simulink model "Robot_1"  (R2023b)
settings: Solver=VariableStepAuto  StartTime=0.0  StopTime=10.0  RelTol=1e-3
settings Model: DataDictionary=Robot_1DD.sldd  Creator=maxju  LastModifiedBy=maxju

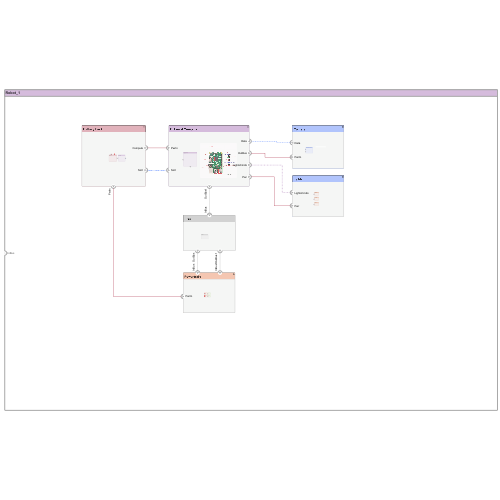
[thumbnail: Simulink's stored preview of the top-level diagram]
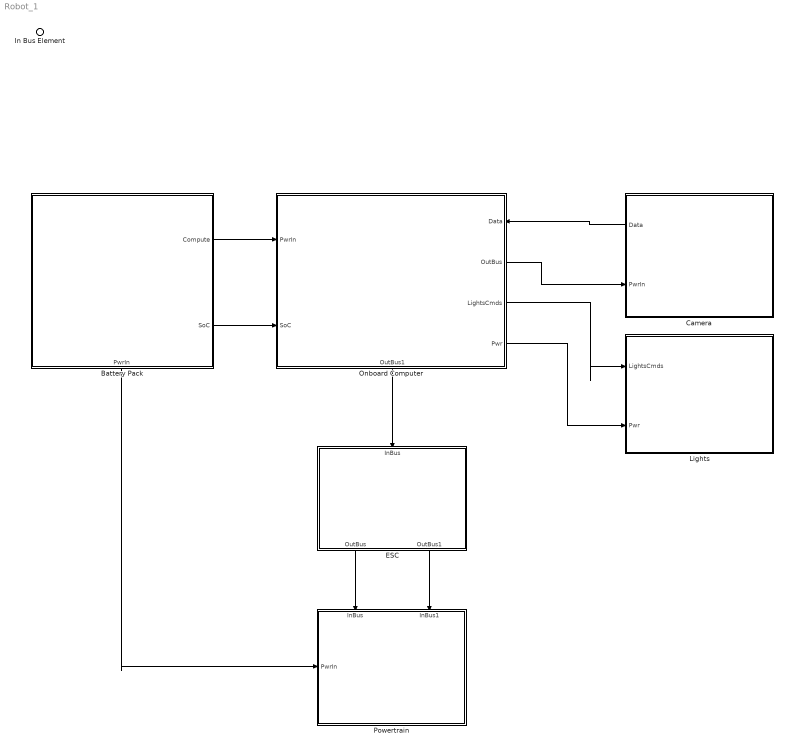
== system Robot_1 ==
  In Bus Element : Inport  PortName=InBus
  Battery Pack : Subsystem
      settings: PortSchema="{\"entries\":[{\"content\":{\"headerSize\":26,\"margin\":15,\"minimumSpacing\":25,\"sides\":[{\"content\":{},\"type\":\"ConnectorPlacement.EquallySpacedRectSide\",\"uuid\":\"346f2912-6369-49a7-a9f0-29be96ed2aab\"},{\"content\":{\"connectorIds\":[\"Out1\",\"Out2\"],\"side\":\"RIGHT\"},\"type\":\"ConnectorPlacement.EquallySpacedRectSide\",\"uuid\":\"c8393630-96ba-47a0-be32-8aed75641cc7\"},{\"content\":{\"side\":\"TOP\"},\"type\":\"ConnectorPlacement.EquallySpacedRectSide\",\"uuid\":\"3ed129fe-5e63-4396-9170-1d52c5d32d40\"},{\"content\":{\"connectorIds\":[\"Out3\"],\"side\":\"BOTTOM\"},\"type\":\"ConnectorPlacement.EquallySpacedRectSide\",\"uuid\":\"1c04906c-6323-40fc-a7b2-3d731de826fc\"}]},\"type\":\"ConnectorPlacement.EquallySpacedConnector\",\"uuid\":\"219e7a86-40fe-4101-a52d-fba84ff528a7\"}],\"packageUris\":[\"http://schema.mathworks.com/mf0/Connector/R2020b\"],\"version\":\"1.0\"}"
  Camera : Subsystem
      settings: PortSchema="{\"entries\":[{\"content\":{\"headerSize\":26,\"margin\":15,\"minimumSpacing\":25,\"sides\":[{\"content\":{\"connectorIds\":[\"Out1\",\"In1\"]},\"type\":\"ConnectorPlacement.EquallySpacedRectSide\",\"uuid\":\"0e3134fb-fb1a-4646-97ad-e2d6271ac93c\"},{\"content\":{\"side\":\"RIGHT\"},\"type\":\"ConnectorPlacement.EquallySpacedRectSide\",\"uuid\":\"f6782e40-1403-4bf9-a42f-252b6616eef0\"},{\"content\":{\"side\":\"TOP\"},\"type\":\"ConnectorPlacement.EquallySpacedRectSide\",\"uuid\":\"161a9c94-3c0d-4f4d-984f-997aeb99b9b4\"}]},\"type\":\"ConnectorPlacement.EquallySpacedConnector\",\"uuid\":\"22acbad8-3a60-4658-bd61-aa1d6af050b7\"}],\"packageUris\":[\"http://schema.mathworks.com/mf0/Connector/R2020b\"],\"version\":\"1.0\"}"
  ESC : Subsystem
      settings: PortSchema="{\"entries\":[{\"content\":{\"headerSize\":26,\"margin\":15,\"minimumSpacing\":25,\"sides\":[{\"content\":{},\"type\":\"ConnectorPlacement.EquallySpacedRectSide\",\"uuid\":\"1141339f-839f-42a9-af72-07ea182886c4\"},{\"content\":{\"side\":\"RIGHT\"},\"type\":\"ConnectorPlacement.EquallySpacedRectSide\",\"uuid\":\"dbe82220-b0cd-4347-8409-f18d181432e5\"},{\"content\":{\"connectorIds\":[\"In1\"],\"side\":\"TOP\"},\"type\":\"ConnectorPlacement.EquallySpacedRectSide\",\"uuid\":\"b87040ad-d69b-40eb-96a3-a12b59f8261a\"},{\"content\":{\"connectorIds\":[\"Out1\",\"Out2\"],\"side\":\"BOTTOM\"},\"type\":\"ConnectorPlacement.EquallySpacedRectSide\",\"uuid\":\"a37703f8-e732-485f-af8e-5cc2f63c328a\"}]},\"type\":\"ConnectorPlacement.EquallySpacedConnector\",\"uuid\":\"cd1bc216-bb56-48d6-9fa3-a849dd38b660\"}],\"packageUris\":[\"http://schema.mathworks.com/mf0/Connector/R2020b\"],\"version\":\"1.0\"}"
  Lights : Subsystem
      settings: PortSchema="{\"entries\":[{\"content\":{\"headerSize\":26,\"margin\":15,\"minimumSpacing\":25,\"sides\":[{\"content\":{\"connectorIds\":[\"In1\",\"In2\"]},\"type\":\"ConnectorPlacement.EquallySpacedRectSide\",\"uuid\":\"346f2912-6369-49a7-a9f0-29be96ed2aab\"},{\"content\":{\"side\":\"RIGHT\"},\"type\":\"ConnectorPlacement.EquallySpacedRectSide\",\"uuid\":\"c8393630-96ba-47a0-be32-8aed75641cc7\"},{\"content\":{\"side\":\"TOP\"},\"type\":\"ConnectorPlacement.EquallySpacedRectSide\",\"uuid\":\"3ed129fe-5e63-4396-9170-1d52c5d32d40\"}]},\"type\":\"ConnectorPlacement.EquallySpacedConnector\",\"uuid\":\"219e7a86-40fe-4101-a52d-fba84ff528a7\"}],\"packageUris\":[\"http://schema.mathworks.com/mf0/Connector/R2020b\"],\"version\":\"1.0\"}"
  Onboard Computer : Subsystem
      settings: PortSchema="{\"entries\":[{\"content\":{\"headerSize\":26,\"margin\":15,\"minimumSpacing\":25,\"sides\":[{\"content\":{\"connectorIds\":[\"In3\",\"In2\"]},\"type\":\"ConnectorPlacement.EquallySpacedRectSide\",\"uuid\":\"346f2912-6369-49a7-a9f0-29be96ed2aab\"},{\"content\":{\"connectorIds\":[\"In1\",\"Out2\",\"Out3\",\"Out4\"],\"side\":\"RIGHT\"},\"type\":\"ConnectorPlacement.EquallySpacedRectSide\",\"uuid\":\"c8393630-96ba-47a0-be32-8aed75641cc7\"},{\"content\":{\"side\":\"TOP\"},\"type\":\"ConnectorPlacement.EquallySpacedRectSide\",\"uuid\":\"3ed129fe-5e63-4396-9170-1d52c5d32d40\"},{\"content\":{\"connectorIds\":[\"Out1\"],\"side\":\"BOTTOM\"},\"type\":\"ConnectorPlacement.EquallySpacedRectSide\",\"uuid\":\"e427383b-7eca-4773-95c8-b4eaaf910589\"}]},\"type\":\"ConnectorPlacement.EquallySpacedConnector\",\"uuid\":\"219e7a86-40fe-4101-a52d-fba84ff528a7\"}],\"packageUris\":[\"http://schema.mathworks.com/mf0/Connector/R2020b\"],\"version\":\"1.0\"}"
  Powertrain : Subsystem
      settings: PortSchema="{\"entries\":[{\"content\":{\"headerSize\":26,\"margin\":15,\"minimumSpacing\":25,\"sides\":[{\"content\":{\"connectorIds\":[\"In3\"]},\"type\":\"ConnectorPlacement.EquallySpacedRectSide\",\"uuid\":\"0e3134fb-fb1a-4646-97ad-e2d6271ac93c\"},{\"content\":{\"side\":\"RIGHT\"},\"type\":\"ConnectorPlacement.EquallySpacedRectSide\",\"uuid\":\"f6782e40-1403-4bf9-a42f-252b6616eef0\"},{\"content\":{\"connectorIds\":[\"In1\",\"In2\"],\"side\":\"TOP\"},\"type\":\"ConnectorPlacement.EquallySpacedRectSide\",\"uuid\":\"161a9c94-3c0d-4f4d-984f-997aeb99b9b4\"},{\"content\":{\"side\":\"BOTTOM\"},\"type\":\"ConnectorPlacement.EquallySpacedRectSide\",\"uuid\":\"0cc85a08-61c2-4dc1-a2c9-a661b3276f19\"}]},\"type\":\"ConnectorPlacement.EquallySpacedConnector\",\"uuid\":\"22acbad8-3a60-4658-bd61-aa1d6af050b7\"}],\"packageUris\":[\"http://schema.mathworks.com/mf0/Connector/R2020b\"],\"version\":\"1.0\"}"
  wires:
  Onboard Computer/1(OutBus1) -> ESC/1(InBus)
  Onboard Computer/3(LightsCmds) -> Lights/1(LightsCmds)
  Onboard Computer/4(Pwr) -> Lights/2(Pwr)
  Onboard Computer/2(OutBus) -> Camera/1(PwrIn)
  Battery Pack/3(PwrIn) -> Powertrain/3(PwrIn)
  Camera/1(Data) -> Onboard Computer/1(Data)
  Battery Pack/1(Compute) -> Onboard Computer/3(PwrIn)
  Battery Pack/2(SoC) -> Onboard Computer/2(SoC)
  ESC/1(OutBus) -> Powertrain/1(InBus)
  ESC/2(OutBus1) -> Powertrain/2(InBus1)

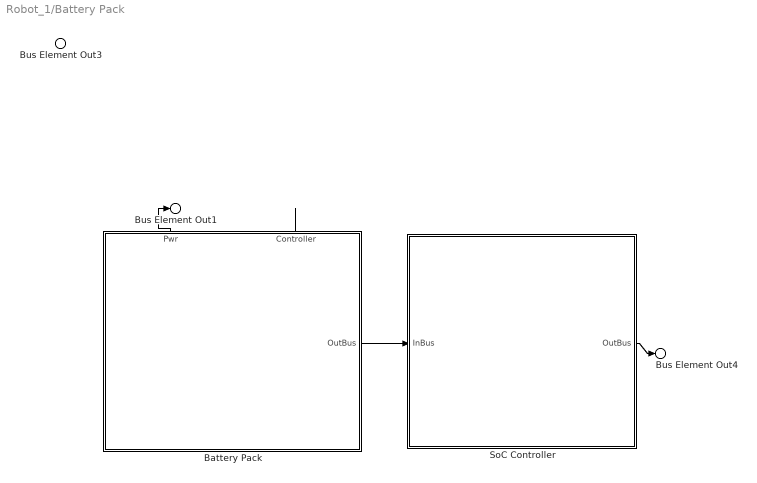
== system Robot_1/Battery Pack ==
  Battery Pack : Subsystem
      settings: PortSchema="{\"entries\":[{\"content\":{\"headerSize\":26,\"margin\":15,\"minimumSpacing\":25,\"sides\":[{\"content\":{},\"type\":\"ConnectorPlacement.EquallySpacedRectSide\",\"uuid\":\"346f2912-6369-49a7-a9f0-29be96ed2aab\"},{\"content\":{\"connectorIds\":[\"Out3\"],\"side\":\"RIGHT\"},\"type\":\"ConnectorPlacement.EquallySpacedRectSide\",\"uuid\":\"c8393630-96ba-47a0-be32-8aed75641cc7\"},{\"content\":{\"connectorIds\":[\"Out1\",\"Out2\"],\"side\":\"TOP\"},\"type\":\"ConnectorPlacement.EquallySpacedRectSide\",\"uuid\":\"3ed129fe-5e63-4396-9170-1d52c5d32d40\"},{\"content\":{\"side\":\"BOTTOM\"},\"type\":\"ConnectorPlacement.EquallySpacedRectSide\",\"uuid\":\"2c97d9a6-c0a8-4633-a49e-90eaf43f5ab4\"}]},\"type\":\"ConnectorPlacement.EquallySpacedConnector\",\"uuid\":\"219e7a86-40fe-4101-a52d-fba84ff528a7\"}],\"packageUris\":[\"http://schema.mathworks.com/mf0/Connector/R2020b\"],\"version\":\"1.0\"}"
  SoC Controller : Subsystem
      settings: PortSchema="{\"entries\":[{\"content\":{\"headerSize\":26,\"margin\":15,\"minimumSpacing\":25,\"sides\":[{\"content\":{\"connectorIds\":[\"In1\"]},\"type\":\"ConnectorPlacement.EquallySpacedRectSide\",\"uuid\":\"cf2231e3-4af8-4ed0-b91c-09d727a3483e\"},{\"content\":{\"connectorIds\":[\"Out1\"],\"side\":\"RIGHT\"},\"type\":\"ConnectorPlacement.EquallySpacedRectSide\",\"uuid\":\"4a4a1d2b-b1e3-400a-adf5-58c88c5da874\"},{\"content\":{\"side\":\"TOP\"},\"type\":\"ConnectorPlacement.EquallySpacedRectSide\",\"uuid\":\"6ce22e2e-ca4b-49c4-85bb-19d8dcc1c047\"}]},\"type\":\"ConnectorPlacement.EquallySpacedConnector\",\"uuid\":\"a895a3e5-be82-4b5e-962f-7a3c361a4de2\"}],\"packageUris\":[\"http://schema.mathworks.com/mf0/Connector/R2020b\"],\"version\":\"1.0\"}"
  Bus Element Out1 : Outport  PortName=Compute  Element=Pwr12V
  Bus Element Out4 : Outport  Port=2  PortName=SoC
  Bus Element Out3 : Outport  Port=3  PortName=PwrIn
  wires:
  Battery Pack/3(OutBus) -> SoC Controller/1(InBus)
  SoC Controller/1(OutBus) -> Bus Element Out4/1
  Battery Pack/1(Pwr) -> Bus Element Out1/1
  Battery Pack/2(Controller) -> ?

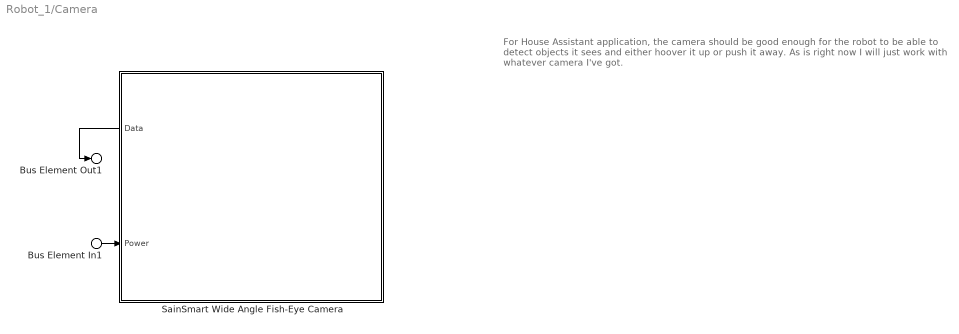
== system Robot_1/Camera ==
  note: For House Assistant application, the camera should be good enough for the robot to be able to detect objects it sees and either hoover it up or push it away.
      | As is right now I will just work with whatever camera I've got.
  Bus Element In1 : Inport  PortName=PwrIn  Element=Pwr6V
  SainSmart Wide Angle Fish-Eye Camera : Subsystem
      settings: PortSchema="{\"entries\":[{\"content\":{\"headerSize\":26,\"margin\":15,\"minimumSpacing\":25,\"sides\":[{\"content\":{\"connectorIds\":[\"Out1\",\"In1\"]},\"type\":\"ConnectorPlacement.EquallySpacedRectSide\",\"uuid\":\"0e3134fb-fb1a-4646-97ad-e2d6271ac93c\"},{\"content\":{\"side\":\"RIGHT\"},\"type\":\"ConnectorPlacement.EquallySpacedRectSide\",\"uuid\":\"f6782e40-1403-4bf9-a42f-252b6616eef0\"},{\"content\":{\"side\":\"TOP\"},\"type\":\"ConnectorPlacement.EquallySpacedRectSide\",\"uuid\":\"161a9c94-3c0d-4f4d-984f-997aeb99b9b4\"}]},\"type\":\"ConnectorPlacement.EquallySpacedConnector\",\"uuid\":\"22acbad8-3a60-4658-bd61-aa1d6af050b7\"}],\"packageUris\":[\"http://schema.mathworks.com/mf0/Connector/R2020b\"],\"version\":\"1.0\"}"
  Bus Element Out1 : Outport  PortName=Data
  wires:
  Bus Element In1/1 -> SainSmart Wide Angle Fish-Eye Camera/1(Power)
  SainSmart Wide Angle Fish-Eye Camera/1(Data) -> Bus Element Out1/1

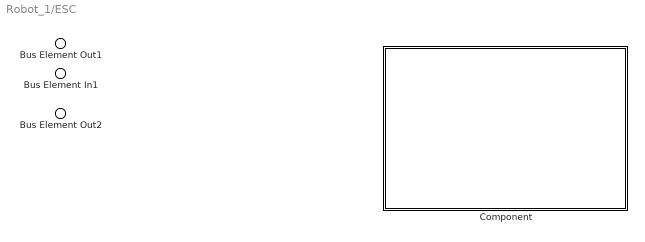
== system Robot_1/ESC ==
  Bus Element In1 : Inport  PortName=InBus
  Component : Subsystem
      settings: PortSchema="{\"entries\":[{\"content\":{\"headerSize\":26,\"margin\":15,\"minimumSpacing\":25,\"sides\":[{\"content\":{},\"type\":\"ConnectorPlacement.EquallySpacedRectSide\",\"uuid\":\"7bd470fa-bce1-4c44-a3a7-0ed7fedee971\"},{\"content\":{\"side\":\"RIGHT\"},\"type\":\"ConnectorPlacement.EquallySpacedRectSide\",\"uuid\":\"b20f4573-2099-47e2-9b7d-c115428c8e1f\"},{\"content\":{\"side\":\"TOP\"},\"type\":\"ConnectorPlacement.EquallySpacedRectSide\",\"uuid\":\"6fe36d19-1289-4062-bd44-05b1c708d213\"}]},\"type\":\"ConnectorPlacement.EquallySpacedConnector\",\"uuid\":\"3a440cc7-8cbc-4545-9d2b-44ca326050ac\"}],\"packageUris\":[\"http://schema.mathworks.com/mf0/Connector/R2020b\"],\"version\":\"1.0\"}"
  Bus Element Out1 : Outport  PortName=OutBus
  Bus Element Out2 : Outport  Port=2  PortName=OutBus1

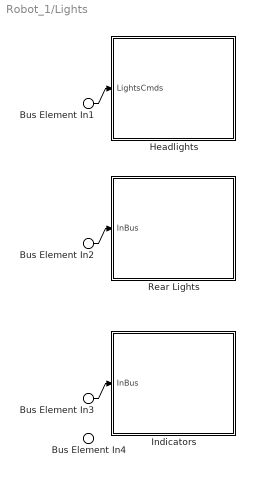
== system Robot_1/Lights ==
  Bus Element In1 : Inport  PortName=LightsCmds  Element=HeadlightsCmds
  Bus Element In2 : Inport  PortName=LightsCmds  Element=RearLightsCmds
  Bus Element In3 : Inport  PortName=LightsCmds  Element=IndicatorsCmds
  Bus Element In4 : Inport  Port=2  PortName=Pwr
  Headlights : Subsystem
      settings: PortSchema="{\"entries\":[{\"content\":{\"headerSize\":26,\"margin\":15,\"minimumSpacing\":25,\"sides\":[{\"content\":{\"connectorIds\":[\"In1\"]},\"type\":\"ConnectorPlacement.EquallySpacedRectSide\",\"uuid\":\"346f2912-6369-49a7-a9f0-29be96ed2aab\"},{\"content\":{\"side\":\"RIGHT\"},\"type\":\"ConnectorPlacement.EquallySpacedRectSide\",\"uuid\":\"c8393630-96ba-47a0-be32-8aed75641cc7\"},{\"content\":{\"side\":\"TOP\"},\"type\":\"ConnectorPlacement.EquallySpacedRectSide\",\"uuid\":\"3ed129fe-5e63-4396-9170-1d52c5d32d40\"}]},\"type\":\"ConnectorPlacement.EquallySpacedConnector\",\"uuid\":\"219e7a86-40fe-4101-a52d-fba84ff528a7\"}],\"packageUris\":[\"http://schema.mathworks.com/mf0/Connector/R2020b\"],\"version\":\"1.0\"}"
  Indicators : Subsystem
      settings: PortSchema="{\"entries\":[{\"content\":{\"headerSize\":26,\"margin\":15,\"minimumSpacing\":25,\"sides\":[{\"content\":{\"connectorIds\":[\"In1\"]},\"type\":\"ConnectorPlacement.EquallySpacedRectSide\",\"uuid\":\"346f2912-6369-49a7-a9f0-29be96ed2aab\"},{\"content\":{\"side\":\"RIGHT\"},\"type\":\"ConnectorPlacement.EquallySpacedRectSide\",\"uuid\":\"c8393630-96ba-47a0-be32-8aed75641cc7\"},{\"content\":{\"side\":\"TOP\"},\"type\":\"ConnectorPlacement.EquallySpacedRectSide\",\"uuid\":\"3ed129fe-5e63-4396-9170-1d52c5d32d40\"}]},\"type\":\"ConnectorPlacement.EquallySpacedConnector\",\"uuid\":\"219e7a86-40fe-4101-a52d-fba84ff528a7\"}],\"packageUris\":[\"http://schema.mathworks.com/mf0/Connector/R2020b\"],\"version\":\"1.0\"}"
  Rear Lights : Subsystem
      settings: PortSchema="{\"entries\":[{\"content\":{\"headerSize\":26,\"margin\":15,\"minimumSpacing\":25,\"sides\":[{\"content\":{\"connectorIds\":[\"In1\"]},\"type\":\"ConnectorPlacement.EquallySpacedRectSide\",\"uuid\":\"346f2912-6369-49a7-a9f0-29be96ed2aab\"},{\"content\":{\"side\":\"RIGHT\"},\"type\":\"ConnectorPlacement.EquallySpacedRectSide\",\"uuid\":\"c8393630-96ba-47a0-be32-8aed75641cc7\"},{\"content\":{\"side\":\"TOP\"},\"type\":\"ConnectorPlacement.EquallySpacedRectSide\",\"uuid\":\"3ed129fe-5e63-4396-9170-1d52c5d32d40\"}]},\"type\":\"ConnectorPlacement.EquallySpacedConnector\",\"uuid\":\"219e7a86-40fe-4101-a52d-fba84ff528a7\"}],\"packageUris\":[\"http://schema.mathworks.com/mf0/Connector/R2020b\"],\"version\":\"1.0\"}"
  wires:
  Bus Element In1/1 -> Headlights/1(LightsCmds)
  Bus Element In2/1 -> Rear Lights/1(InBus)
  Bus Element In3/1 -> Indicators/1(InBus)

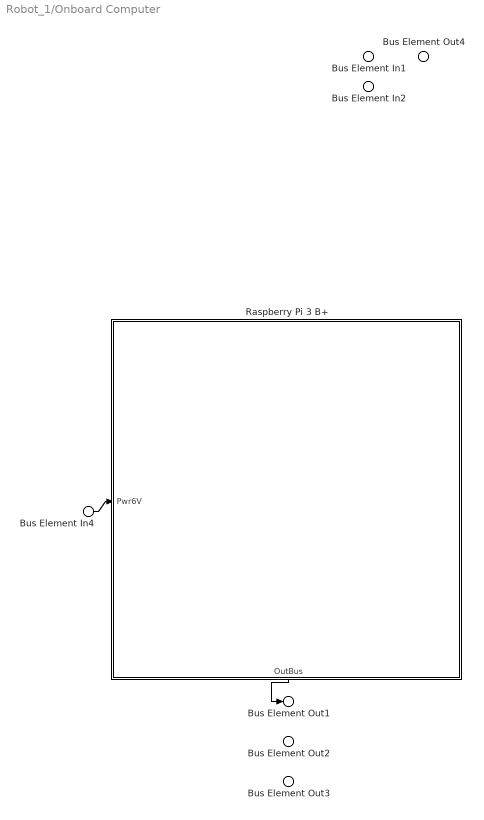
== system Robot_1/Onboard Computer ==
  Bus Element In1 : Inport  PortName=Data
  Bus Element In2 : Inport  Port=2  PortName=SoC
  Bus Element In4 : Inport  Port=3  PortName=PwrIn  Element=Pwr12V
  Raspberry Pi 3 B+ : Stateflow chart  TreatAsAtomicUnit=on
      settings: PortSchema="{\"entries\":[{\"content\":{\"headerSize\":26,\"margin\":15,\"minimumSpacing\":25,\"sides\":[{\"content\":{\"connectorIds\":[\"In1\"]},\"type\":\"ConnectorPlacement.EquallySpacedRectSide\",\"uuid\":\"0e3134fb-fb1a-4646-97ad-e2d6271ac93c\"},{\"content\":{\"side\":\"RIGHT\"},\"type\":\"ConnectorPlacement.EquallySpacedRectSide\",\"uuid\":\"f6782e40-1403-4bf9-a42f-252b6616eef0\"},{\"content\":{\"side\":\"TOP\"},\"type\":\"ConnectorPlacement.EquallySpacedRectSide\",\"uuid\":\"161a9c94-3c0d-4f4d-984f-997aeb99b9b4\"},{\"content\":{\"connectorIds\":[\"Out1\"],\"side\":\"BOTTOM\"},\"type\":\"ConnectorPlacement.EquallySpacedRectSide\",\"uuid\":\"bf1e25a0-eb6f-4642-8c09-fa933b1d8126\"}]},\"type\":\"ConnectorPlacement.EquallySpacedConnector\",\"uuid\":\"22acbad8-3a60-4658-bd61-aa1d6af050b7\"}],\"packageUris\":[\"http://schema.mathworks.com/mf0/Connector/R2020b\"],\"version\":\"1.0\"}"
  Bus Element Out4 : Outport  PortName=OutBus1
  Bus Element Out1 : Outport  Port=2  PortName=OutBus  Element=Pwr6V
  Bus Element Out2 : Outport  Port=3  PortName=LightsCmds
  Bus Element Out3 : Outport  Port=4  PortName=Pwr
  wires:
  Bus Element In4/1 -> Raspberry Pi 3 B+/1(Pwr6V)
  Raspberry Pi 3 B+/1(OutBus) -> Bus Element Out1/1

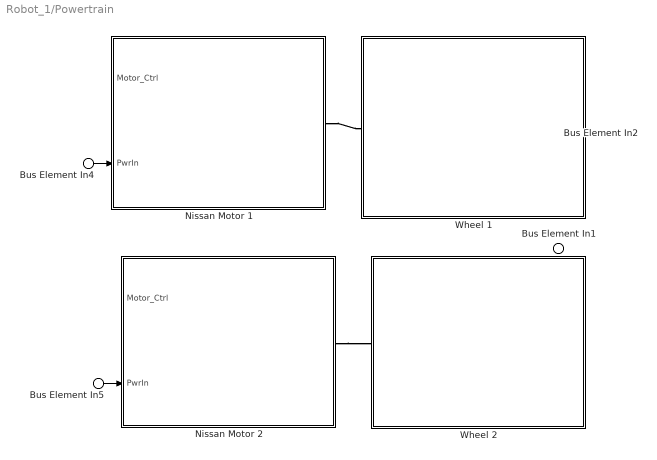
== system Robot_1/Powertrain ==
  Bus Element In1 : Inport  PortName=InBus
  Bus Element In2 : Inport  Port=2  PortName=InBus1
  Bus Element In4 : Inport  Port=3  PortName=PwrIn
  Bus Element In5 : Inport  Port=3  PortName=PwrIn
  Nissan Motor 1 : Subsystem
      settings: PortSchema="{\"entries\":[{\"content\":{\"headerSize\":26,\"margin\":15,\"minimumSpacing\":25,\"sides\":[{\"content\":{\"connectorIds\":[\"In1\",\"In2\"]},\"type\":\"ConnectorPlacement.EquallySpacedRectSide\",\"uuid\":\"346f2912-6369-49a7-a9f0-29be96ed2aab\"},{\"content\":{\"connectorIds\":[\"RConn1\"],\"side\":\"RIGHT\"},\"type\":\"ConnectorPlacement.EquallySpacedRectSide\",\"uuid\":\"c8393630-96ba-47a0-be32-8aed75641cc7\"},{\"content\":{\"side\":\"TOP\"},\"type\":\"ConnectorPlacement.EquallySpacedRectSide\",\"uuid\":\"3ed129fe-5e63-4396-9170-1d52c5d32d40\"}]},\"type\":\"ConnectorPlacement.EquallySpacedConnector\",\"uuid\":\"219e7a86-40fe-4101-a52d-fba84ff528a7\"}],\"packageUris\":[\"http://schema.mathworks.com/mf0/Connector/R2020b\"],\"version\":\"1.0\"}"
  Nissan Motor 2 : Subsystem
      settings: PortSchema="{\"entries\":[{\"content\":{\"headerSize\":26,\"margin\":15,\"minimumSpacing\":25,\"sides\":[{\"content\":{\"connectorIds\":[\"In1\",\"In2\"]},\"type\":\"ConnectorPlacement.EquallySpacedRectSide\",\"uuid\":\"346f2912-6369-49a7-a9f0-29be96ed2aab\"},{\"content\":{\"connectorIds\":[\"RConn1\"],\"side\":\"RIGHT\"},\"type\":\"ConnectorPlacement.EquallySpacedRectSide\",\"uuid\":\"c8393630-96ba-47a0-be32-8aed75641cc7\"},{\"content\":{\"side\":\"TOP\"},\"type\":\"ConnectorPlacement.EquallySpacedRectSide\",\"uuid\":\"3ed129fe-5e63-4396-9170-1d52c5d32d40\"}]},\"type\":\"ConnectorPlacement.EquallySpacedConnector\",\"uuid\":\"219e7a86-40fe-4101-a52d-fba84ff528a7\"}],\"packageUris\":[\"http://schema.mathworks.com/mf0/Connector/R2020b\"],\"version\":\"1.0\"}"
  Wheel 1 : Subsystem
      settings: PortSchema="{\"entries\":[{\"content\":{\"headerSize\":26,\"margin\":15,\"minimumSpacing\":25,\"sides\":[{\"content\":{\"connectorIds\":[\"LConn1\"]},\"type\":\"ConnectorPlacement.EquallySpacedRectSide\",\"uuid\":\"dc8ac33d-fe92-43e0-a9c9-04d1e5888cff\"},{\"content\":{\"side\":\"RIGHT\"},\"type\":\"ConnectorPlacement.EquallySpacedRectSide\",\"uuid\":\"e43c357d-5116-4011-b344-dfb9e111863c\"},{\"content\":{\"side\":\"TOP\"},\"type\":\"ConnectorPlacement.EquallySpacedRectSide\",\"uuid\":\"f49f6d22-f7fb-4476-908a-f2ab6c48c2d4\"}]},\"type\":\"ConnectorPlacement.EquallySpacedConnector\",\"uuid\":\"ff34b972-cd2d-47ab-a722-1d2e1f6984bd\"}],\"packageUris\":[\"http://schema.mathworks.com/mf0/Connector/R2020b\"],\"version\":\"1.0\"}"
  Wheel 2 : Subsystem
      settings: PortSchema="{\"entries\":[{\"content\":{\"headerSize\":26,\"margin\":15,\"minimumSpacing\":25,\"sides\":[{\"content\":{\"connectorIds\":[\"LConn1\"]},\"type\":\"ConnectorPlacement.EquallySpacedRectSide\",\"uuid\":\"dc8ac33d-fe92-43e0-a9c9-04d1e5888cff\"},{\"content\":{\"side\":\"RIGHT\"},\"type\":\"ConnectorPlacement.EquallySpacedRectSide\",\"uuid\":\"e43c357d-5116-4011-b344-dfb9e111863c\"},{\"content\":{\"side\":\"TOP\"},\"type\":\"ConnectorPlacement.EquallySpacedRectSide\",\"uuid\":\"f49f6d22-f7fb-4476-908a-f2ab6c48c2d4\"}]},\"type\":\"ConnectorPlacement.EquallySpacedConnector\",\"uuid\":\"ff34b972-cd2d-47ab-a722-1d2e1f6984bd\"}],\"packageUris\":[\"http://schema.mathworks.com/mf0/Connector/R2020b\"],\"version\":\"1.0\"}"
  wires:
  ? -> Nissan Motor 1/1(Motor_Ctrl)
  ? -> Nissan Motor 2/1(Motor_Ctrl)
  Bus Element In4/1 -> Nissan Motor 1/2(PwrIn)
  Bus Element In5/1 -> Nissan Motor 2/2(PwrIn)
  connections:
  Nissan Motor 2/RConn1 -- Wheel 2/LConn1
  Nissan Motor 1/RConn1 -- Wheel 1/LConn1

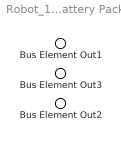
== system Robot_1/Battery Pack/Battery Pack ==
  Bus Element Out1 : Outport  PortName=Pwr
  Bus Element Out2 : Outport  Port=2  PortName=Controller
  Bus Element Out3 : Outport  Port=3  PortName=OutBus

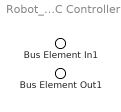
== system Robot_1/Battery Pack/SoC Controller ==
  Bus Element In1 : Inport  PortName=InBus
  Bus Element Out1 : Outport  PortName=OutBus

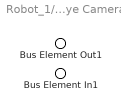
== system Robot_1/Camera/SainSmart Wide Angle Fish-Eye Camera ==
  Bus Element In1 : Inport  PortName=Power
  Bus Element Out1 : Outport  PortName=Data

== system Robot_1/ESC/Component ==

== system Robot_1/Lights/Headlights ==
  Bus Element In1 : Inport  PortName=LightsCmds

== system Robot_1/Lights/Indicators ==
  Bus Element In1 : Inport  PortName=InBus

== system Robot_1/Lights/Rear Lights ==
  Bus Element In1 : Inport  PortName=InBus

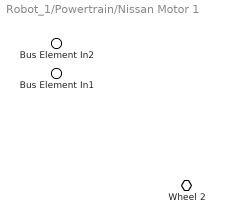
== system Robot_1/Powertrain/Nissan Motor 1 ==
  Bus Element In1 : Inport  PortName=Motor_Ctrl
  Bus Element In2 : Inport  Port=2  PortName=PwrIn
  Wheel 2 : PMIOPort  Side=Right

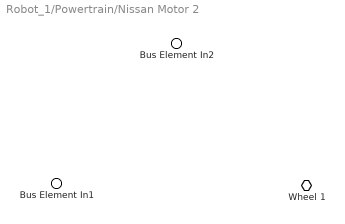
== system Robot_1/Powertrain/Nissan Motor 2 ==
  Bus Element In2 : Inport  PortName=Motor_Ctrl
  Bus Element In1 : Inport  Port=2  PortName=PwrIn
  Wheel 1 : PMIOPort  Side=Right

== system Robot_1/Powertrain/Wheel 1 ==
  Wheel 2 : PMIOPort  Side=Left

== system Robot_1/Powertrain/Wheel 2 ==
  Wheel 1 : PMIOPort  Side=Left

== stateflow chart Robot_1/Onboard Computer/Raspberry Pi 3 B+ ==
  data: Pwr6V input Bus: Pwr; OutBus output
